simulink model "w2_warplab_trigger_proc"  (Simulink 7.7)
settings: Solver=ode45  StartTime=0.0  StopTime=1000  RelTol=1e-3
InitFcn:
  | w2_warplab_trigger_proc_init
StartFcn:
  | w2_warplab_trigger_proc_init
undefined symbols (not defined in the file or in its folder): gcbh, xlBlockLoadCallback, xlGetNormalizedPeriod
libraries: xbsIndex_r4 x819, simulink x1
(part 2 of 6)

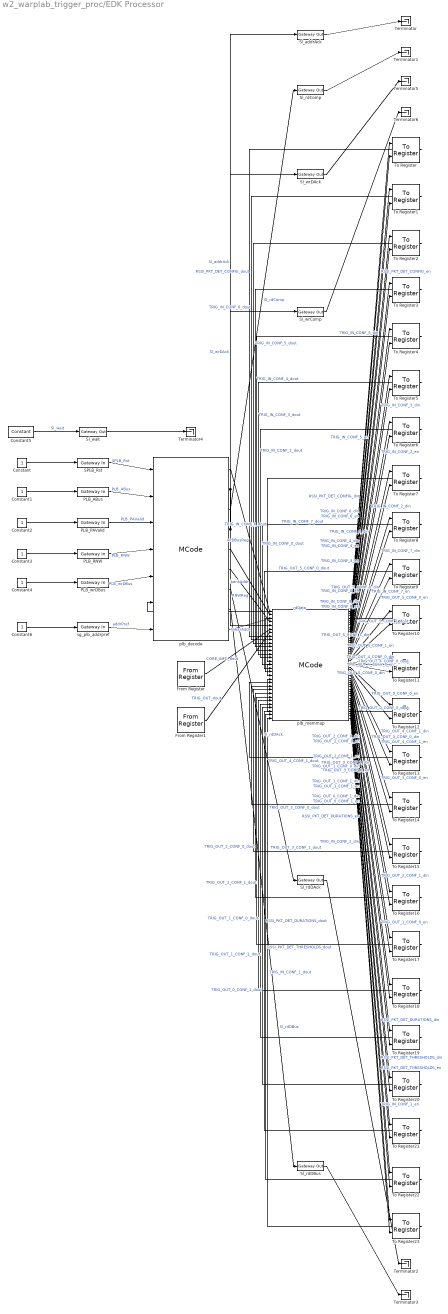
== system w2_warplab_trigger_proc/EDK Processor ==
  Constant{,1..4,6} (6 alike) : Constant
  Constant5 : xbsIndex_r4/Constant  const=0  gui_display_data_type=Fixed-point  arith_type=Unsigned  n_bits=1  bin_pt=0  preci_type=Single  exp_width=8  frac_width=24  explicit_period=on  period=xlGetNormalizedPeriod()  equ=P=C  opselect=C  inp2=PCIN>>17  opr=+  inp1=P  carry=CIN  dbl_ovrd=off  block_type=constant
  From Register : xbsIndex_r4/From Register  shared_memory_name='CORE_INFO'  init=0  period=xlGetNormalizedPeriod()  ownership=Owned and initialized elsewhere  gui_display_data_type=Fixed-point  arith_type=Unsigned  n_bits=24  bin_pt=0  preci_type=Single  dbl_ovrd=off  block_type=fromreg
      settings: AttributesFormatString=<< %<shared_memory_name> >>  infoedit="Register block that reads data to a shared memory register.  Delay of one sample period."
  From Register1 : xbsIndex_r4/From Register  shared_memory_name='TRIG_OUT'  init=0  period=xlGetNormalizedPeriod()  ownership=Owned and initialized elsewhere  gui_display_data_type=Fixed-point  arith_type=Unsigned  n_bits=6  bin_pt=0  preci_type=Single  dbl_ovrd=off  block_type=fromreg
      settings: AttributesFormatString=<< %<shared_memory_name> >>  infoedit="Register block that reads data to a shared memory register.  Delay of one sample period."
  PLB_ABus : xbsIndex_r4/Gateway In  gui_display_data_type=Fixed-point  arith_type=Unsigned  n_bits=32  bin_pt=0  preci_type=Single  exp_width=8  frac_width=24  quantization="Round  (unbiased: +/- Inf)"  overflow=Saturate  period=xlGetNormalizedPeriod()  dbl_ovrd=off  timing_constraint=None  locs_specified=off  LOCs={}  UseAsADC=off  ADCChannel='1'  inherit_from_input=off  hdl_port=on  block_type=gatewayin
      settings: sginterface={'Xilinx'=>{'jtaghwcosim'=>{'non_memory_mapped_port'=>'PLB_ABus'}},'iopad'=>{'constraint'=>'#'}}
  PLB_PAValid : xbsIndex_r4/Gateway In  gui_display_data_type=Fixed-point  arith_type=Unsigned  n_bits=1  bin_pt=0  preci_type=Single  exp_width=8  frac_width=24  quantization="Round  (unbiased: +/- Inf)"  overflow=Saturate  period=xlGetNormalizedPeriod()  dbl_ovrd=off  timing_constraint=None  locs_specified=off  LOCs={}  UseAsADC=off  ADCChannel='1'  inherit_from_input=off  hdl_port=on  block_type=gatewayin
      settings: sginterface={'Xilinx'=>{'jtaghwcosim'=>{'non_memory_mapped_port'=>'PLB_PAValid'}},'iopad'=>{'constraint'=>'#'}}
  PLB_RNW : xbsIndex_r4/Gateway In  gui_display_data_type=Fixed-point  arith_type=Unsigned  n_bits=1  bin_pt=0  preci_type=Single  exp_width=8  frac_width=24  quantization="Round  (unbiased: +/- Inf)"  overflow=Saturate  period=xlGetNormalizedPeriod()  dbl_ovrd=off  timing_constraint=None  locs_specified=off  LOCs={}  UseAsADC=off  ADCChannel='1'  inherit_from_input=off  hdl_port=on  block_type=gatewayin
      settings: sginterface={'Xilinx'=>{'jtaghwcosim'=>{'non_memory_mapped_port'=>'PLB_RNW'}},'iopad'=>{'constraint'=>'#'}}
  PLB_wrDBus : xbsIndex_r4/Gateway In  gui_display_data_type=Fixed-point  arith_type=Unsigned  n_bits=32  bin_pt=0  preci_type=Single  exp_width=8  frac_width=24  quantization="Round  (unbiased: +/- Inf)"  overflow=Saturate  period=xlGetNormalizedPeriod()  dbl_ovrd=off  timing_constraint=None  locs_specified=off  LOCs={}  UseAsADC=off  ADCChannel='1'  inherit_from_input=off  hdl_port=on  block_type=gatewayin
      settings: sginterface={'Xilinx'=>{'jtaghwcosim'=>{'non_memory_mapped_port'=>'PLB_wrDBus'}},'iopad'=>{'constraint'=>'#'}}
  SPLB_Rst : xbsIndex_r4/Gateway In  gui_display_data_type=Fixed-point  arith_type=Unsigned  n_bits=1  bin_pt=0  preci_type=Single  exp_width=8  frac_width=24  quantization="Round  (unbiased: +/- Inf)"  overflow=Saturate  period=xlGetNormalizedPeriod()  dbl_ovrd=off  timing_constraint=None  locs_specified=off  LOCs={}  UseAsADC=off  ADCChannel='1'  inherit_from_input=off  hdl_port=on  block_type=gatewayin
      settings: sginterface={'Xilinx'=>{'jtaghwcosim'=>{'non_memory_mapped_port'=>'SPLB_Rst'}},'iopad'=>{'constraint'=>'#'}}
  Sl_addrAck : xbsIndex_r4/Gateway Out  inherit_from_input=off  hdl_port=on  timing_constraint=None  locs_specified=off  LOCs={}  UseAsDAC=off  DACChannel='1'  block_type=gatewayout
      settings: sginterface={'Xilinx'=>{'jtaghwcosim'=>{'non_memory_mapped_port'=>'Sl_addrAck'}},'iopad'=>{'constraint'=>'#'}}
  Sl_rdComp : xbsIndex_r4/Gateway Out  inherit_from_input=off  hdl_port=on  timing_constraint=None  locs_specified=off  LOCs={}  UseAsDAC=off  DACChannel='1'  block_type=gatewayout
      settings: sginterface={'Xilinx'=>{'jtaghwcosim'=>{'non_memory_mapped_port'=>'Sl_rdComp'}},'iopad'=>{'constraint'=>'#'}}
  Sl_rdDAck : xbsIndex_r4/Gateway Out  inherit_from_input=off  hdl_port=on  timing_constraint=None  locs_specified=off  LOCs={}  UseAsDAC=off  DACChannel='1'  block_type=gatewayout
      settings: sginterface={'Xilinx'=>{'jtaghwcosim'=>{'non_memory_mapped_port'=>'Sl_rdDAck'}},'iopad'=>{'constraint'=>'#'}}
  Sl_rdDBus : xbsIndex_r4/Gateway Out  inherit_from_input=off  hdl_port=on  timing_constraint=None  locs_specified=off  LOCs={}  UseAsDAC=off  DACChannel='1'  block_type=gatewayout
      settings: sginterface={'Xilinx'=>{'jtaghwcosim'=>{'non_memory_mapped_port'=>'Sl_rdDBus'}},'iopad'=>{'constraint'=>'#'}}
  Sl_wait : xbsIndex_r4/Gateway Out  inherit_from_input=off  hdl_port=on  timing_constraint=None  locs_specified=off  LOCs={}  UseAsDAC=off  DACChannel='1'  block_type=gatewayout
      settings: sginterface={'Xilinx'=>{'jtaghwcosim'=>{'non_memory_mapped_port'=>'Sl_wait'}},'iopad'=>{'constraint'=>'#'}}
  Sl_wrComp : xbsIndex_r4/Gateway Out  inherit_from_input=off  hdl_port=on  timing_constraint=None  locs_specified=off  LOCs={}  UseAsDAC=off  DACChannel='1'  block_type=gatewayout
      settings: sginterface={'Xilinx'=>{'jtaghwcosim'=>{'non_memory_mapped_port'=>'Sl_wrComp'}},'iopad'=>{'constraint'=>'#'}}
  Sl_wrDAck : xbsIndex_r4/Gateway Out  inherit_from_input=off  hdl_port=on  timing_constraint=None  locs_specified=off  LOCs={}  UseAsDAC=off  DACChannel='1'  block_type=gatewayout
      settings: sginterface={'Xilinx'=>{'jtaghwcosim'=>{'non_memory_mapped_port'=>'Sl_wrDAck'}},'iopad'=>{'constraint'=>'#'}}
  Terminator{,1..6} (7 alike) : Terminator
  To Register : xbsIndex_r4/To Register  shared_memory_name='RSSI_PKT_DET_CONFIG'  init=0  ownership=Owned and initialized elsewhere  explicit_data_type=on  gui_display_data_type=Fixed-point  arith_type=Unsigned  n_bits=32  bin_pt=0  preci_type=Single  dbl_ovrd=off  block_type=toreg
      settings: AttributesFormatString=<< %<shared_memory_name> >>  infoedit="Register block that writes data to a shared memory register.  Delay of one sample period."
  To Register1 : xbsIndex_r4/To Register  shared_memory_name='TRIG_IN_CONF_6'  init=0  ownership=Owned and initialized elsewhere  explicit_data_type=on  gui_display_data_type=Fixed-point  arith_type=Unsigned  n_bits=32  bin_pt=0  preci_type=Single  dbl_ovrd=off  block_type=toreg
      settings: AttributesFormatString=<< %<shared_memory_name> >>  infoedit="Register block that writes data to a shared memory register.  Delay of one sample period."
  To Register10 : xbsIndex_r4/To Register  shared_memory_name='TRIG_OUT_5_CONF_1'  init=0  ownership=Owned and initialized elsewhere  explicit_data_type=on  gui_display_data_type=Fixed-point  arith_type=Unsigned  n_bits=32  bin_pt=0  preci_type=Single  dbl_ovrd=off  block_type=toreg
      settings: AttributesFormatString=<< %<shared_memory_name> >>  infoedit="Register block that writes data to a shared memory register.  Delay of one sample period."
  To Register11 : xbsIndex_r4/To Register  shared_memory_name='TRIG_OUT_4_CONF_0'  init=0  ownership=Owned and initialized elsewhere  explicit_data_type=on  gui_display_data_type=Fixed-point  arith_type=Unsigned  n_bits=32  bin_pt=0  preci_type=Single  dbl_ovrd=off  block_type=toreg
      settings: AttributesFormatString=<< %<shared_memory_name> >>  infoedit="Register block that writes data to a shared memory register.  Delay of one sample period."
  To Register12 : xbsIndex_r4/To Register  shared_memory_name='TRIG_OUT_0_CONF_0'  init=0  ownership=Owned and initialized elsewhere  explicit_data_type=on  gui_display_data_type=Fixed-point  arith_type=Unsigned  n_bits=32  bin_pt=0  preci_type=Single  dbl_ovrd=off  block_type=toreg
      settings: AttributesFormatString=<< %<shared_memory_name> >>  infoedit="Register block that writes data to a shared memory register.  Delay of one sample period."
  To Register13 : xbsIndex_r4/To Register  shared_memory_name='TRIG_OUT_4_CONF_1'  init=0  ownership=Owned and initialized elsewhere  explicit_data_type=on  gui_display_data_type=Fixed-point  arith_type=Unsigned  n_bits=32  bin_pt=0  preci_type=Single  dbl_ovrd=off  block_type=toreg
      settings: AttributesFormatString=<< %<shared_memory_name> >>  infoedit="Register block that writes data to a shared memory register.  Delay of one sample period."
  To Register14 : xbsIndex_r4/To Register  shared_memory_name='TRIG_OUT_3_CONF_0'  init=0  ownership=Owned and initialized elsewhere  explicit_data_type=on  gui_display_data_type=Fixed-point  arith_type=Unsigned  n_bits=32  bin_pt=0  preci_type=Single  dbl_ovrd=off  block_type=toreg
      settings: AttributesFormatString=<< %<shared_memory_name> >>  infoedit="Register block that writes data to a shared memory register.  Delay of one sample period."
  To Register15 : xbsIndex_r4/To Register  shared_memory_name='TRIG_OUT_3_CONF_1'  init=0  ownership=Owned and initialized elsewhere  explicit_data_type=on  gui_display_data_type=Fixed-point  arith_type=Unsigned  n_bits=32  bin_pt=0  preci_type=Single  dbl_ovrd=off  block_type=toreg
      settings: AttributesFormatString=<< %<shared_memory_name> >>  infoedit="Register block that writes data to a shared memory register.  Delay of one sample period."
  To Register16 : xbsIndex_r4/To Register  shared_memory_name='TRIG_OUT_2_CONF_0'  init=0  ownership=Owned and initialized elsewhere  explicit_data_type=on  gui_display_data_type=Fixed-point  arith_type=Unsigned  n_bits=32  bin_pt=0  preci_type=Single  dbl_ovrd=off  block_type=toreg
      settings: AttributesFormatString=<< %<shared_memory_name> >>  infoedit="Register block that writes data to a shared memory register.  Delay of one sample period."
  To Register17 : xbsIndex_r4/To Register  shared_memory_name='TRIG_OUT_2_CONF_1'  init=0  ownership=Owned and initialized elsewhere  explicit_data_type=on  gui_display_data_type=Fixed-point  arith_type=Unsigned  n_bits=32  bin_pt=0  preci_type=Single  dbl_ovrd=off  block_type=toreg
      settings: AttributesFormatString=<< %<shared_memory_name> >>  infoedit="Register block that writes data to a shared memory register.  Delay of one sample period."
  To Register18 : xbsIndex_r4/To Register  shared_memory_name='TRIG_OUT_1_CONF_0'  init=0  ownership=Owned and initialized elsewhere  explicit_data_type=on  gui_display_data_type=Fixed-point  arith_type=Unsigned  n_bits=32  bin_pt=0  preci_type=Single  dbl_ovrd=off  block_type=toreg
      settings: AttributesFormatString=<< %<shared_memory_name> >>  infoedit="Register block that writes data to a shared memory register.  Delay of one sample period."
  To Register19 : xbsIndex_r4/To Register  shared_memory_name='TRIG_OUT_1_CONF_1'  init=0  ownership=Owned and initialized elsewhere  explicit_data_type=on  gui_display_data_type=Fixed-point  arith_type=Unsigned  n_bits=32  bin_pt=0  preci_type=Single  dbl_ovrd=off  block_type=toreg
      settings: AttributesFormatString=<< %<shared_memory_name> >>  infoedit="Register block that writes data to a shared memory register.  Delay of one sample period."
  To Register2 : xbsIndex_r4/To Register  shared_memory_name='TRIG_IN_CONF_5'  init=0  ownership=Owned and initialized elsewhere  explicit_data_type=on  gui_display_data_type=Fixed-point  arith_type=Unsigned  n_bits=32  bin_pt=0  preci_type=Single  dbl_ovrd=off  block_type=toreg
      settings: AttributesFormatString=<< %<shared_memory_name> >>  infoedit="Register block that writes data to a shared memory register.  Delay of one sample period."
  To Register20 : xbsIndex_r4/To Register  shared_memory_name='TRIG_OUT_0_CONF_1'  init=0  ownership=Owned and initialized elsewhere  explicit_data_type=on  gui_display_data_type=Fixed-point  arith_type=Unsigned  n_bits=32  bin_pt=0  preci_type=Single  dbl_ovrd=off  block_type=toreg
      settings: AttributesFormatString=<< %<shared_memory_name> >>  infoedit="Register block that writes data to a shared memory register.  Delay of one sample period."
  To Register21 : xbsIndex_r4/To Register  shared_memory_name='RSSI_PKT_DET_DURATIONS'  init=0  ownership=Owned and initialized elsewhere  explicit_data_type=on  gui_display_data_type=Fixed-point  arith_type=Unsigned  n_bits=32  bin_pt=0  preci_type=Single  dbl_ovrd=off  block_type=toreg
      settings: AttributesFormatString=<< %<shared_memory_name> >>  infoedit="Register block that writes data to a shared memory register.  Delay of one sample period."
  To Register22 : xbsIndex_r4/To Register  shared_memory_name='RSSI_PKT_DET_THRESHOLDS'  init=0  ownership=Owned and initialized elsewhere  explicit_data_type=on  gui_display_data_type=Fixed-point  arith_type=Unsigned  n_bits=32  bin_pt=0  preci_type=Single  dbl_ovrd=off  block_type=toreg
      settings: AttributesFormatString=<< %<shared_memory_name> >>  infoedit="Register block that writes data to a shared memory register.  Delay of one sample period."
  To Register23 : xbsIndex_r4/To Register  shared_memory_name='TRIG_IN_CONF_1'  init=0  ownership=Owned and initialized elsewhere  explicit_data_type=on  gui_display_data_type=Fixed-point  arith_type=Unsigned  n_bits=32  bin_pt=0  preci_type=Single  dbl_ovrd=off  block_type=toreg
      settings: AttributesFormatString=<< %<shared_memory_name> >>  infoedit="Register block that writes data to a shared memory register.  Delay of one sample period."
  To Register3 : xbsIndex_r4/To Register  shared_memory_name='TRIG_IN_CONF_4'  init=0  ownership=Owned and initialized elsewhere  explicit_data_type=on  gui_display_data_type=Fixed-point  arith_type=Unsigned  n_bits=32  bin_pt=0  preci_type=Single  dbl_ovrd=off  block_type=toreg
      settings: AttributesFormatString=<< %<shared_memory_name> >>  infoedit="Register block that writes data to a shared memory register.  Delay of one sample period."
  To Register4 : xbsIndex_r4/To Register  shared_memory_name='TRIG_IN_CONF_3'  init=0  ownership=Owned and initialized elsewhere  explicit_data_type=on  gui_display_data_type=Fixed-point  arith_type=Unsigned  n_bits=32  bin_pt=0  preci_type=Single  dbl_ovrd=off  block_type=toreg
      settings: AttributesFormatString=<< %<shared_memory_name> >>  infoedit="Register block that writes data to a shared memory register.  Delay of one sample period."
  To Register5 : xbsIndex_r4/To Register  shared_memory_name='TRIG_IN_CONF_2'  init=0  ownership=Owned and initialized elsewhere  explicit_data_type=on  gui_display_data_type=Fixed-point  arith_type=Unsigned  n_bits=32  bin_pt=0  preci_type=Single  dbl_ovrd=off  block_type=toreg
      settings: AttributesFormatString=<< %<shared_memory_name> >>  infoedit="Register block that writes data to a shared memory register.  Delay of one sample period."
  To Register6 : xbsIndex_r4/To Register  shared_memory_name='TRIG_IN_CONF_0'  init=0  ownership=Owned and initialized elsewhere  explicit_data_type=on  gui_display_data_type=Fixed-point  arith_type=Unsigned  n_bits=32  bin_pt=0  preci_type=Single  dbl_ovrd=off  block_type=toreg
      settings: AttributesFormatString=<< %<shared_memory_name> >>  infoedit="Register block that writes data to a shared memory register.  Delay of one sample period."
  To Register7 : xbsIndex_r4/To Register  shared_memory_name='TRIG_IN_CONF_8'  init=0  ownership=Owned and initialized elsewhere  explicit_data_type=on  gui_display_data_type=Fixed-point  arith_type=Unsigned  n_bits=32  bin_pt=0  preci_type=Single  dbl_ovrd=off  block_type=toreg
      settings: AttributesFormatString=<< %<shared_memory_name> >>  infoedit="Register block that writes data to a shared memory register.  Delay of one sample period."
  To Register8 : xbsIndex_r4/To Register  shared_memory_name='TRIG_IN_CONF_7'  init=0  ownership=Owned and initialized elsewhere  explicit_data_type=on  gui_display_data_type=Fixed-point  arith_type=Unsigned  n_bits=32  bin_pt=0  preci_type=Single  dbl_ovrd=off  block_type=toreg
      settings: AttributesFormatString=<< %<shared_memory_name> >>  infoedit="Register block that writes data to a shared memory register.  Delay of one sample period."
  To Register9 : xbsIndex_r4/To Register  shared_memory_name='TRIG_OUT_5_CONF_0'  init=0  ownership=Owned and initialized elsewhere  explicit_data_type=on  gui_display_data_type=Fixed-point  arith_type=Unsigned  n_bits=32  bin_pt=0  preci_type=Single  dbl_ovrd=off  block_type=toreg
      settings: AttributesFormatString=<< %<shared_memory_name> >>  infoedit="Register block that writes data to a shared memory register.  Delay of one sample period."
  plb_decode : xbsIndex_r4/MCode  mfname=xlmax  explicit_period=off  period=1  dbl_ovrd=off  enable_stdout=off  enable_debug=off  mfilecontent=|  suppress_output=on  defparams={}  hide_port_list={}  block_type=mcode
      | function [wrDBusReg, addrAck, rdComp, wrDAck, bankAddr, RNWReg, rdDAck, rdDBus, linearAddr] = plb_bus_decode(plbRst, plbABus, plbPAValid, plbRNW, plbWrDBus, rdData, addrPref)
      | 
      | % constant variables (TODO: should pass from outside)
      | ADDRPREF_LEN = 20;
      | BANKADDR_LEN = 2;
      | LINEARADDR_LEN = 8;
      | ABUS_LEN = 32;
      | DBUS_LEN = 32;
      | 
      | % declare and initialize persistent variables
      | % register input bus signals
      | persistent plbRstReg_, plbRstReg_ = xl_state(0, {xlBoolean});
      | persistent plbABusReg_, plbABusReg_ = xl_state(0, {xlUnsigned, ABUS_LEN, 0});
      | persistent plbPAValidReg_, plbPAValidReg_ = xl_state(0, {xlBoolean});
      | persistent plbRNWReg_, plbRNWReg_ = xl_state(0, {xlUnsigned, 1, 0});
      | persistent plbWrDBusReg_, plbWrDBusReg_ = xl_state(0, {xlUnsigned, DBUS_LEN, 0});
      | 
      | % ===== rest of the outputs =====
      | 
      | bankAddr   = xl_slice(plbABusReg_, 2+BANKADDR_LEN+LINEARADDR_LEN-1, 2+LINEARADDR_LEN);
      | linearAddr = xl_slice(plbABusReg_, 2+LINEARADDR_LEN-1, 2);
      | RNWReg = plbRNWReg_;
      | wrDBusReg = plbWrDBusReg_;
      | 
      | % ===== p_select =====
      | 
      | % register PAValid
      | persistent aValidReg, aValidReg = xl_state(0, {xlBoolean});
      | aValidReg = plbPAValidReg_;
      | 
      | % extract and register the address prefix
      | addrPref_in = xl_slice(plbABusReg_, xl_nbits(plbABusReg_)-1, xl_nbits(plbABusReg_)-ADDRPREF_LEN);
      | if addrPref_in == addrPref
      |     ps1 = true;
      | else 
      |     ps1 = false;
      | end 
      | 
      | persistent ps1Reg, ps1Reg = xl_state(0, ps1);
      | ps1Reg = ps1;
      | 
      | ps = xl_and(ps1Reg, aValidReg);
      | 
      | % ===== addrAck =====
      | 
      | % register ps
      | persistent psReg, psReg = xl_state(0, ps);
      | 
      | addrAck = xfix({xlUnsigned, 1, 0}, xl_and(xl_not(plbRstReg_), ps, xl_not(psReg)));
      | 
      | psReg = ps;
      | 
      | % ===== rdComp, rd/wr DAck =====
      |  
      | rdComp1 = xfix({xlUnsigned, 1, 0}, xl_and(addrAck, RNWReg));
      | 
      | NUM_rdCompDelay = 3;
      | persistent rdCompDelay, rdCompDelay = xl_state(zeros(1, NUM_rdCompDelay), rdComp1, NUM_rdCompDelay);
      | rdComp2 = rdCompDelay.back;
      | rdCompDelay.push_front_pop_back(rdComp1);
      | 
      | persistent rdCompReg, rdCompReg = xl_state(0, rdComp1);
      | rdComp = rdCompReg;
      | rdCompReg = rdComp2;
      | 
      | persistent rdDAckReg, rdDAckReg = xl_state(0, rdComp1);
      | rdDAck = rdDAckReg;
      | rdDAckReg = rdComp;
      | 
      | persistent wrDAckReg, wrDAckReg = xl_state(0, addrAck);
      | wrDAck = wrDAckReg;
      | wrDAckReg = xl_and(addrAck, xl_not(RNWReg));
      | 
      | % ===== rdDBus =====
      | 
      | rdSel = xl_or(rdComp2, rdComp);
      | 
      | if rdSel == 1
      |     rdDBus1 = rdData;
      | else
      |     rdDBus1 = 0;
      | end % if
      | 
      | persistent rdDBusReg, rdDBusReg = xl_state(0, rdDBus1);
      | rdDBus = rdDBusReg;
      | rdDBusReg = rdDBus1;
      | 
      | % rdDBus = xl_concat(rdDBus32, rdDBus32);
      | % rdDBus = rdDBus32;
      | 
      | % ===== update the persistent variables =====
      | 
      | plbRstReg_ = plbRst;
      | plbABusReg_ = plbABus;
      | plbPAValidReg_ = plbPAValid;
      | plbRNWReg_ = plbRNW;
      | plbWrDBusReg_ = xl_slice(plbWrDBus, DBUS_LEN-1, 0);
  plb_memmap : xbsIndex_r4/MCode  mfname=xlmax  explicit_period=off  period=1  dbl_ovrd=off  enable_stdout=off  enable_debug=off  mfilecontent=|  suppress_output=on  defparams={}  hide_port_list={}  block_type=mcode
      | function [read_bank_out, sm_RSSI_PKT_DET_CONFIG_din, sm_RSSI_PKT_DET_CONFIG_en, sm_TRIG_IN_CONF_6_din, sm_TRIG_IN_CONF_6_en, sm_TRIG_IN_CONF_5_din, sm_TRIG_IN_CONF_5_en, sm_TRIG_IN_CONF_4_din, sm_TRIG_IN_CONF_4_en, sm_TRIG_IN_CONF_3_din, sm_TRIG_IN_CONF_3_en, sm_TRIG_IN_CONF_2_din, sm_TRIG_IN_CONF_2_en, sm_TRIG_IN_CONF_0_din, sm_TRIG_IN_CONF_0_en, sm_TRIG_IN_CONF_8_din, sm_TRIG_IN_CONF_8_en, sm_TRIG_IN_CONF_7_din, sm_TRIG_IN_CONF_7_en, sm_TRIG_OUT_5_CONF_0_din, sm_TRIG_OUT_5_CONF_0_en, sm_TRIG_OUT_5_CONF_1_din, sm_TRIG_OUT_5_CONF_1_en, sm_TRIG_OUT_4_CONF_0_din, sm_TRIG_OUT_4_CONF_0_en, sm_TRIG_OUT_0_CONF_0_din, sm_TRIG_OUT_0_CONF_0_en, sm_TRIG_OUT_4_CONF_1_din, sm_TRIG_OUT_4_CONF_1_en, sm_TRIG_OUT_3_CONF_0_din, sm_TRIG_OUT_3_CONF_0_en, sm_TRIG_OUT_3_CONF_1_din, sm_TRIG_OUT_3_CONF_1_en, sm_TRIG_OUT_2_CONF_0_din, sm_TRIG_OUT_2_CONF_0_en, sm_TRIG_OUT_2_CONF_1_din, sm_TRIG_OUT_2_CONF_1_en, sm_TRIG_OUT_1_CONF_0_din, sm_TRIG_OUT_1_CONF_0_en, sm_TRIG_OUT_1_CONF_1_din, sm_TRIG_OUT_1_CONF_1_en, sm_TRIG_OUT_0_CONF_1_din, sm_TRIG_OUT_0_CONF_1_en, sm_RSSI_PKT_DET_DURATIONS_din, sm_RSSI_PKT_DET_DURATIONS_en, sm_RSSI_PKT_DET_THRESHOLDS_din, sm_RSSI_PKT_DET_THRESHOLDS_en, sm_TRIG_IN_CONF_1_din, sm_TRIG_IN_CONF_1_en] = plb_memmap(wrDBus, bankAddr, linearAddr, RNWReg, addrAck, sm_CORE_INFO, sm_TRIG_OUT, sm_RSSI_PKT_DET_CONFIG, sm_TRIG_IN_CONF_6, sm_TRIG_IN_CONF_5, sm_TRIG_IN_CONF_4, sm_TRIG_IN_CONF_3, sm_TRIG_IN_CONF_2, sm_TRIG_IN_CONF_0, sm_TRIG_IN_CONF_8, sm_TRIG_IN_CONF_7, sm_TRIG_OUT_5_CONF_0, sm_TRIG_OUT_5_CONF_1, sm_TRIG_OUT_4_CONF_0, sm_TRIG_OUT_0_CONF_0, sm_TRIG_OUT_4_CONF_1, sm_TRIG_OUT_3_CONF_0, sm_TRIG_OUT_3_CONF_1, sm_TRIG_OUT_2_CONF_0, sm_TRIG_OUT_2_CONF_1, sm_TRIG_OUT_1_CONF_0, sm_TRIG_OUT_1_CONF_1, sm_TRIG_OUT_0_CONF_1, sm_RSSI_PKT_DET_DURATIONS, sm_RSSI_PKT_DET_THRESHOLDS, sm_TRIG_IN_CONF_1)
      | 
      | 
      | % connvert the input data to UFix_32_0 (the bus data type)
      | % 'From Register' blocks
      | % sm_CORE_INFO_bus = xfix({xlUnsigned, 32, 0}, 0);
      | sm_CORE_INFO_bus = xl_force(sm_CORE_INFO, xlUnsigned, 0);
      | 
      | % sm_TRIG_OUT_bus = xfix({xlUnsigned, 32, 0}, 0);
      | sm_TRIG_OUT_bus = xl_force(sm_TRIG_OUT, xlUnsigned, 0);
      | 
      | % 'To Register' blocks
      | 
      | % sm_RSSI_PKT_DET_CONFIG_dout = xfix({xlUnsigned, 32, 0}, 0);
      | sm_RSSI_PKT_DET_CONFIG_dout = xl_force(sm_RSSI_PKT_DET_CONFIG, xlUnsigned, 0);
      | 
      | % sm_TRIG_IN_CONF_6_dout = xfix({xlUnsigned, 32, 0}, 0);
      | sm_TRIG_IN_CONF_6_dout = xl_force(sm_TRIG_IN_CONF_6, xlUnsigned, 0);
      | 
      | % sm_TRIG_IN_CONF_5_dout = xfix({xlUnsigned, 32, 0}, 0);
      | sm_TRIG_IN_CONF_5_dout = xl_force(sm_TRIG_IN_CONF_5, xlUnsigned, 0);
      | 
      | % sm_TRIG_IN_CONF_4_dout = xfix({xlUnsigned, 32, 0}, 0);
      | sm_TRIG_IN_CONF_4_dout = xl_force(sm_TRIG_IN_CONF_4, xlUnsigned, 0);
      | 
      | % sm_TRIG_IN_CONF_3_dout = xfix({xlUnsigned, 32, 0}, 0);
      | sm_TRIG_IN_CONF_3_dout = xl_force(sm_TRIG_IN_CONF_3, xlUnsigned, 0);
      | 
      | % sm_TRIG_IN_CONF_2_dout = xfix({xlUnsigned, 32, 0}, 0);
      | sm_TRIG_IN_CONF_2_dout = xl_force(sm_TRIG_IN_CONF_2, xlUnsigned, 0);
      | 
      | % sm_TRIG_IN_CONF_0_dout = xfix({xlUnsigned, 32, 0}, 0);
      | sm_TRIG_IN_CONF_0_dout = xl_force(sm_TRIG_IN_CONF_0, xlUnsigned, 0);
      | 
      | % sm_TRIG_IN_CONF_8_dout = xfix({xlUnsigned, 32, 0}, 0);
      | sm_TRIG_IN_CONF_8_dout = xl_force(sm_TRIG_IN_CONF_8, xlUnsigned, 0);
      | 
      | % sm_TRIG_IN_CONF_7_dout = xfix({xlUnsigned, 32, 0}, 0);
      | sm_TRIG_IN_CONF_7_dout = xl_force(sm_TRIG_IN_CONF_7, xlUnsigned, 0);
      | 
      | % sm_TRIG_OUT_5_CONF_0_dout = xfix({xlUnsigned, 32, 0}, 0);
      | sm_TRIG_OUT_5_CONF_0_dout = xl_force(sm_TRIG_OUT_5_CONF_0, xlUnsigned, 0);
      | 
      | % sm_TRIG_OUT_5_CONF_1_dout = xfix({xlUnsigned, 32, 0}, 0);
      | sm_TRIG_OUT_5_CONF_1_dout = xl_force(sm_TRIG_OUT_5_CONF_1, xlUnsigned, 0);
      | 
      | % sm_TRIG_OUT_4_CONF_0_dout = xfix({xlUnsigned, 32, 0}, 0);
      | sm_TRIG_OUT_4_CONF_0_dout = xl_force(sm_TRIG_OUT_4_CONF_0, xlUnsigned, 0);
      | 
      | % sm_TRIG_OUT_0_CONF_0_dout = xfix({xlUnsigned, 32, 0}, 0);
      | sm_TRIG_OUT_0_CONF_0_dout = xl_force(sm_TRIG_OUT_0_CONF_0, xlUnsigned, 0);
      | 
      | % sm_TRIG_OUT_4_CONF_1_dout = xfix({xlUnsigned, 32, 0}, 0);
      | sm_TRIG_OUT_4_CONF_1_dout = xl_force(sm_TRIG_OUT_4_CONF_1, xlUnsigned, 0);
      | 
      | % sm_TRIG_OUT_3_CONF_0_dout = xfix({xlUnsigned, 32, 0}, 0);
      | sm_TRIG_OUT_3_CONF_0_dout = xl_force(sm_TRIG_OUT_3_CONF_0, xlUnsigned, 0);
      | 
      | % sm_TRIG_OUT_3_CONF_1_dout = xfix({xlUnsigned, 32, 0}, 0);
      | sm_TRIG_OUT_3_CONF_1_dout = xl_force(sm_TRIG_OUT_3_CONF_1, xlUnsigned, 0);
      | 
      | % sm_TRIG_OUT_2_CONF_0_dout = xfix({xlUnsigned, 32, 0}, 0);
      | sm_TRIG_OUT_2_CONF_0_dout = xl_force(sm_TRIG_OUT_2_CONF_0, xlUnsigned, 0);
      | 
      | % sm_TRIG_OUT_2_CONF_1_dout = xfix({xlUnsigned, 32, 0}, 0);
      | sm_TRIG_OUT_2_CONF_1_dout = xl_force(sm_TRIG_OUT_2_CONF_1, xlUnsigned, 0);
      | 
      | % sm_TRIG_OUT_1_CONF_0_dout = xfix({xlUnsigned, 32, 0}, 0);
      | sm_TRIG_OUT_1_CONF_0_dout = xl_force(sm_TRIG_OUT_1_CONF_0, xlUnsigned, 0);
      | 
      | % sm_TRIG_OUT_1_CONF_1_dout = xfix({xlUnsigned, 32, 0}, 0);
      | sm_TRIG_OUT_1_CONF_1_dout = xl_force(sm_TRIG_OUT_1_CONF_1, xlUnsigned, 0);
      | 
      | % sm_TRIG_OUT_0_CONF_1_dout = xfix({xlUnsigned, 32, 0}, 0);
      | sm_TRIG_OUT_0_CONF_1_dout = xl_force(sm_TRIG_OUT_0_CONF_1, xlUnsigned, 0);
      | 
      | % sm_RSSI_PKT_DET_DURATIONS_dout = xfix({xlUnsigned, 32, 0}, 0);
      | sm_RSSI_PKT_DET_DURATIONS_dout = xl_force(sm_RSSI_PKT_DET_DURATIONS, xlUnsigned, 0);
      | 
      | % sm_RSSI_PKT_DET_THRESHOLDS_dout = xfix({xlUnsigned, 32, 0}, 0);
      | sm_RSSI_PKT_DET_THRESHOLDS_dout = xl_force(sm_RSSI_PKT_DET_THRESHOLDS, xlUnsigned, 0);
      | 
      | % sm_TRIG_IN_CONF_1_dout = xfix({xlUnsigned, 32, 0}, 0);
      | sm_TRIG_IN_CONF_1_dout = xl_force(sm_TRIG_IN_CONF_1, xlUnsigned, 0);
      | 
      | 
      | % 'From FIFO' blocks
      | % 'To FIFO' blocks
      | % 'Shared Memory' blocks
      | 
      | % 'dout' ports of 'From Register' blocks
      | 
      | % registered register mux output
      | persistent reg_bank_out_reg; reg_bank_out_reg = xl_state(0, {xlUnsigned, 32, 0});
      | reg_bank_out = reg_bank_out_reg;
      | 
      | if linearAddr == 24
      |     reg_bank_out_reg = sm_CORE_INFO_bus;
      | elseif linearAddr == 25
      |     reg_bank_out_reg = sm_TRIG_OUT_bus;
      | elseif linearAddr == 0
      |     reg_bank_out_reg = sm_RSSI_PKT_DET_CONFIG_dout;
      | elseif linearAddr == 1
      |     reg_bank_out_reg = sm_TRIG_IN_CONF_6_dout;
      | elseif linearAddr == 2
      |     reg_bank_out_reg = sm_TRIG_IN_CONF_5_dout;
      | elseif linearAddr == 3
      |     reg_bank_out_reg = sm_TRIG_IN_CONF_4_dout;
      | elseif linearAddr == 4
      |     reg_bank_out_reg = sm_TRIG_IN_CONF_3_dout;
      | elseif linearAddr == 5
      |     reg_bank_out_reg = sm_TRIG_IN_CONF_2_dout;
      | elseif linearAddr == 6
      |     reg_bank_out_reg = sm_TRIG_IN_CONF_0_dout;
      | elseif linearAddr == 7
      |     reg_bank_out_reg = sm_TRIG_IN_CONF_8_dout;
      | elseif linearAddr == 8
      |     reg_bank_out_reg = sm_TRIG_IN_CONF_7_dout;
      | elseif linearAddr == 9
      |     reg_bank_out_reg = sm_TRIG_OUT_5_CONF_0_dout;
      | elseif linearAddr == 10
      |     reg_bank_out_reg = sm_TRIG_OUT_5_CONF_1_dout;
      | elseif linearAddr == 11
      |     reg_bank_out_reg = sm_TRIG_OUT_4_CONF_0_dout;
      | elseif linearAddr == 12
      |     reg_bank_out_reg = sm_TRIG_OUT_0_CONF_0_dout;
      | elseif linearAddr == 13
      |     reg_bank_out_reg = sm_TRIG_OUT_4_CONF_1_dout;
      | elseif linearAddr == 14
      |     reg_bank_out_reg = sm_TRIG_OUT_3_CONF_0_dout;
      | elseif linearAddr == 15
      |     reg_bank_out_reg = sm_TRIG_OUT_3_CONF_1_dout;
      | elseif linearAddr == 16
      |     reg_bank_out_reg = sm_TRIG_OUT_2_CONF_0_dout;
      | elseif linearAddr == 17
      |     reg_bank_out_reg = sm_TRIG_OUT_2_CONF_1_dout;
      | elseif linearAddr == 18
      |     reg_bank_out_reg = sm_TRIG_OUT_1_CONF_0_dout;
      | elseif linearAddr == 19
      |     reg_bank_out_reg = sm_TRIG_OUT_1_CONF_1_dout;
      | elseif linearAddr == 20
      |     reg_bank_out_reg = sm_TRIG_OUT_0_CONF_1_dout;
      | elseif linearAddr == 21
      |     reg_bank_out_reg = sm_RSSI_PKT_DET_DURATIONS_dout;
      | elseif linearAddr == 22
      |     reg_bank_out_reg = sm_RSSI_PKT_DET_THRESHOLDS_dout;
      | elseif linearAddr == 23
      |     reg_bank_out_reg = sm_TRIG_IN_CONF_1_dout;
      | 
      | end
      | 
      | 
      | % 'From FIFO' and 'To FIFO' blocks
      | 
      | 
      | 
      | 
      | 
      | opCode = xl_concat(addrAck, RNWReg, bankAddr, linearAddr);
      | 
      | % 'Shared Memory' blocks
      | 
      | 
      | 
      | 
      | 
      | % 'din' ports of 'Shared Memory' blocks
      | 
      | 
      | % 'we' ports of 'Shared Memory' blocks
      | 
      | 
      | % 'addr' ports of 'Shared Memory' blocks
      | 
      | 
      | % 're' ports of 'From FIFO' blocks
      | 
      | 
      | % 'en' ports of 'To Register' blocks
      | if opCode == xl_concat(xfix({xlUnsigned, 4, 0}, 10), ...
      |                        xfix({xlUnsigned, xl_nbits(linearAddr), 0}, 0))
      |     sm_RSSI_PKT_DET_CONFIG_en = true;
      | else
      |     sm_RSSI_PKT_DET_CONFIG_en = false;
      | end
      | if opCode == xl_concat(xfix({xlUnsigned, 4, 0}, 10), ...
      |                        xfix({xlUnsigned, xl_nbits(linearAddr), 0}, 1))
      |     sm_TRIG_IN_CONF_6_en = true;
      | else
      |     sm_TRIG_IN_CONF_6_en = false;
      | end
      | if opCode == xl_concat(xfix({xlUnsigned, 4, 0}, 10), ...
      |                        xfix({xlUnsigned, xl_nbits(linearAddr), 0}, 2))
      |     sm_TRIG_IN_CONF_5_en = true;
      | else
      |     sm_TRIG_IN_CONF_5_en = false;
      | end
      | if opCode == xl_concat(xfix({xlUnsigned, 4, 0}, 10), ...
      |                        xfix({xlUnsigned, xl_nbits(linearAddr), 0}, 3))
      |     sm_TRIG_IN_CONF_4_en = true;
      | else
      |     sm_TRIG_IN_CONF_4_en = false;
      | end
      | if opCode == xl_concat(xfix({xlUnsigned, 4, 0}, 10), ...
      |                        xfix({xlUnsigned, xl_nbits(linearAddr), 0}, 4))
      |     sm_TRIG_IN_CONF_3_en = true;
      | else
      |     sm_TRIG_IN_CONF_3_en = false;
      | end
      | if opCode == xl_concat(xfix({xlUnsigned, 4, 0}, 10), ...
      |                        xfix({xlUnsigned, xl_nbits(linearAddr), 0}, 5))
      |     sm_TRIG_IN_CONF_2_en = true;
      | else
      |     sm_TRIG_IN_CONF_2_en = false;
      | end
      | if opCode == xl_concat(xfix({xlUnsigned, 4, 0}, 10), ...
      |                        xfix({xlUnsigned, xl_nbits(linearAddr), 0}, 6))
      |     sm_TRIG_IN_CONF_0_en = true;
      | else
      |     sm_TRIG_IN_CONF_0_en = false;
      | end
      | if opCode == xl_concat(xfix({xlUnsigned, 4, 0}, 10), ...
      |                        xfix({xlUnsigned, xl_nbits(linearAddr), 0}, 7))
      |     sm_TRIG_IN_CONF_8_en = true;
      | else
      |     sm_TRIG_IN_CONF_8_en = false;
      | end
      | if opCode == xl_concat(xfix({xlUnsigned, 4, 0}, 10), ...
      |                        xfix({xlUnsigned, xl_nbits(linearAddr), 0}, 8))
      |     sm_TRIG_IN_CONF_7_en = true;
      | else
      |     sm_TRIG_IN_CONF_7_en = false;
      | end
      | if opCode == xl_concat(xfix({xlUnsigned, 4, 0}, 10), ...
      |                        xfix({xlUnsigned, xl_nbits(linearAddr), 0}, 9))
      |     sm_TRIG_OUT_5_CONF_0_en = true;
      | else
      |     sm_TRIG_OUT_5_CONF_0_en = false;
      | end
      | if opCode == xl_concat(xfix({xlUnsigned, 4, 0}, 10), ...
      |                        xfix({xlUnsigned, xl_nbits(linearAddr), 0}, 10))
      |     sm_TRIG_OUT_5_CONF_1_en = true;
      | else
      |     sm_TRIG_OUT_5_CONF_1_en = false;
      | end
      | if opCode == xl_concat(xfix({xlUnsigned, 4, 0}, 10), ...
      |                        xfix({xlUnsigned, xl_nbits(linearAddr), 0}, 11))
      |     sm_TRIG_OUT_4_CONF_0_en = true;
      | else
      |     sm_TRIG_OUT_4_CONF_0_en = false;
      | end
      | if opCode == xl_concat(xfix({xlUnsigned, 4, 0}, 10), ...
      |                        xfix({xlUnsigned, xl_nbits(linearAddr), 0}, 12))
      |     sm_TRIG_OUT_0_CONF_0_en = true;
      | else
      |     sm_TRIG_OUT_0_CONF_0_en = false;
      | end
      | if opCode == xl_concat(xfix({xlUnsigned, 4, 0}, 10), ...
      |                        xfix({xlUnsigned, xl_nbits(linearAddr), 0}, 13))
      |     sm_TRIG_OUT_4_CONF_1_en = true;
      | else
      |     sm_TRIG_OUT_4_CONF_1_en = false;
      | end
      | if opCode == xl_concat(xfix({xlUnsigned, 4, 0}, 10), ...
      |                        xfix({xlUnsigned, xl_nbits(linearAddr), 0}, 14))
      |     sm_TRIG_OUT_3_CONF_0_en = true;
      | else
      |     sm_TRIG_OUT_3_CONF_0_en = false;
      | end
      | if opCode == xl_concat(xfix({xlUnsigned, 4, 0}, 10), ...
      |                        xfix({xlUnsigned, xl_nbits(linearAddr), 0}, 15))
      |     sm_TRIG_OUT_3_CONF_1_en = true;
      | else
      |     sm_TRIG_OUT_3_CONF_1_en = false;
      | end
      | if opCode == xl_concat(xfix({xlUnsigned, 4, 0}, 10), ...
      |                        xfix({xlUnsigned, xl_nbits(linearAddr), 0}, 16))
      |     sm_TRIG_OUT_2_CONF_0_en = true;
      | else
      |     sm_TRIG_OUT_2_CONF_0_en = false;
      | end
      | if opCode == xl_concat(xfix({xlUnsigned, 4, 0}, 10), ...
      |                        xfix({xlUnsigned, xl_nbits(linearAddr), 0}, 17))
      |     sm_TRIG_OUT_2_CONF_1_en = true;
      | else
      |     sm_TRIG_OUT_2_CONF_1_en = false;
      | end
      | if opCode == xl_concat(xfix({xlUnsigned, 4, 0}, 10), ...
      |                        xfix({xlUnsigned, xl_nbits(linearAddr), 0}, 18))
      |     sm_TRIG_OUT_1_CONF_0_en = true;
      | else
      |     sm_TRIG_OUT_1_CONF_0_en = false;
      | end
      | if opCode == xl_concat(xfix({xlUnsigned, 4, 0}, 10), ...
      |                        xfix({xlUnsigned, xl_nbits(linearAddr), 0}, 19))
      |     sm_TRIG_OUT_1_CONF_1_en = true;
      | else
      |     sm_TRIG_OUT_1_CONF_1_en = false;
      | end
      | if opCode == xl_concat(xfix({xlUnsigned, 4, 0}, 10), ...
      |                        xfix({xlUnsigned, xl_nbits(linearAddr), 0}, 20))
      |     sm_TRIG_OUT_0_CONF_1_en = true;
      | else
      |     sm_TRIG_OUT_0_CONF_1_en = false;
      | end
      | if opCode == xl_concat(xfix({xlUnsigned, 4, 0}, 10), ...
      |                        xfix({xlUnsigned, xl_nbits(linearAddr), 0}, 21))
      |     sm_RSSI_PKT_DET_DURATIONS_en = true;
      | else
      |     sm_RSSI_PKT_DET_DURATIONS_en = false;
      | end
      | if opCode == xl_concat(xfix({xlUnsigned, 4, 0}, 10), ...
      |                        xfix({xlUnsigned, xl_nbits(linearAddr), 0}, 22))
      |     sm_RSSI_PKT_DET_THRESHOLDS_en = true;
      | else
      |     sm_RSSI_PKT_DET_THRESHOLDS_en = false;
      | end
      | if opCode == xl_concat(xfix({xlUnsigned, 4, 0}, 10), ...
      |                        xfix({xlUnsigned, xl_nbits(linearAddr), 0}, 23))
      |     sm_TRIG_IN_CONF_1_en = true;
      | else
      |     sm_TRIG_IN_CONF_1_en = false;
      | end
      | 
      | 
      | % 'din' ports of 'To FIFO' blocks
      | 
      | 
      | % 'we' ports of 'To FIFO' blocks
      | 
      | 
      | % 'din' ports of 'To Register' blocks
      | sm_RSSI_PKT_DET_CONFIG_din = xl_force(xl_slice(wrDBus, 32 - 1, 0), ...
      |                                  xlUnsigned, ...
      |                                  0);
      | sm_TRIG_IN_CONF_6_din = xl_force(xl_slice(wrDBus, 32 - 1, 0), ...
      |                                  xlUnsigned, ...
      |                                  0);
      | sm_TRIG_IN_CONF_5_din = xl_force(xl_slice(wrDBus, 32 - 1, 0), ...
      |                                  xlUnsigned, ...
      |                                  0);
      | sm_TRIG_IN_CONF_4_din = xl_force(xl_slice(wrDBus, 32 - 1, 0), ...
      |                                  xlUnsigned, ...
      |                                  0);
      | sm_TRIG_IN_CONF_3_din = xl_force(xl_slice(wrDBus, 32 - 1, 0), ...
      |                                  xlUnsigned, ...
      |                                  0);
      | sm_TRIG_IN_CONF_2_din = xl_force(xl_slice(wrDBus, 32 - 1, 0), ...
      |                                  xlUnsigned, ...
      |                                  0);
      | sm_TRIG_IN_CONF_0_din = xl_force(xl_slice(wrDBus, 32 - 1, 0), ...
      |                                  xlUnsigned, ...
      |                                  0);
      | sm_TRIG_IN_CONF_8_din = xl_force(xl_slice(wrDBus, 32 - 1, 0), ...
      |                                  xlUnsigned, ...
      |                                  0);
      | sm_TRIG_IN_CONF_7_din = xl_force(xl_slice(wrDBus, 32 - 1, 0), ...
      |                                  xlUnsigned, ...
      |                                  0);
      | sm_TRIG_OUT_5_CONF_0_din = xl_force(xl_slice(wrDBus, 32 - 1, 0), ...
      |                                  xlUnsigned, ...
      |                                  0);
      | sm_TRIG_OUT_5_CONF_1_din = xl_force(xl_slice(wrDBus, 32 - 1, 0), ...
      |                                  xlUnsigned, ...
      |                                  0);
      | sm_TRIG_OUT_4_CONF_0_din = xl_force(xl_slice(wrDBus, 32 - 1, 0), ...
      |                                  xlUnsigned, ...
      |                                  0);
      | sm_TRIG_OUT_0_CONF_0_din = xl_force(xl_slice(wrDBus, 32 - 1, 0), ...
      |                                  xlUnsigned, ...
      |                                  0);
      | sm_TRIG_OUT_4_CONF_1_din = xl_force(xl_slice(wrDBus, 32 - 1, 0), ...
      |                                  xlUnsigned, ...
      |                                  0);
      | sm_TRIG_OUT_3_CONF_0_din = xl_force(xl_slice(wrDBus, 32 - 1, 0), ...
      |                                  xlUnsigned, ...
      |                                  0);
      | sm_TRIG_OUT_3_CONF_1_din = xl_force(xl_slice(wrDBus, 32 - 1, 0), ...
      |                                  xlUnsigned, ...
      |                                  0);
      | sm_TRIG_OUT_2_CONF_0_din = xl_force(xl_slice(wrDBus, 32 - 1, 0), ...
      |                                  xlUnsigned, ...
      |                                  0);
      | sm_TRIG_OUT_2_CONF_1_din = xl_force(xl_slice(wrDBus, 32 - 1, 0), ...
      |                                  xlUnsigned, ...
      |                                  0);
      | sm_TRIG_OUT_1_CONF_0_din = xl_force(xl_slice(wrDBus, 32 - 1, 0), ...
      |                                  xlUnsigned, ...
      |                                  0);
      | sm_TRIG_OUT_1_CONF_1_din = xl_force(xl_slice(wrDBus, 32 - 1, 0), ...
      |                                  xlUnsigned, ...
      |                                  0);
      | sm_TRIG_OUT_0_CONF_1_din = xl_force(xl_slice(wrDBus, 32 - 1, 0), ...
      |                                  xlUnsigned, ...
      |                                  0);
      | sm_RSSI_PKT_DET_DURATIONS_din = xl_force(xl_slice(wrDBus, 32 - 1, 0), ...
      |                                  xlUnsigned, ...
      |                                  0);
      | sm_RSSI_PKT_DET_THRESHOLDS_din = xl_force(xl_slice(wrDBus, 32 - 1, 0), ...
      |                                  xlUnsigned, ...
      |                                  0);
      | sm_TRIG_IN_CONF_1_din = xl_force(xl_slice(wrDBus, 32 - 1, 0), ...
      |                                  xlUnsigned, ...
      |                                  0);
      | 
      | 
      | persistent read_bank_out_reg; read_bank_out_reg = xl_state(0, {xlUnsigned, 32, 0});
      | read_bank_out = read_bank_out_reg;
      | 
      | persistent bankAddr_reg; bankAddr_reg = xl_state(0, bankAddr);
      | 
      | if bankAddr_reg == 0
      |     % Bank 0: Shared Memories
      |     read_bank_out_reg = 0;
      | elseif bankAddr_reg == 1
      |     % Bank 1: From/To FIFOs
      |     read_bank_out_reg =  0;
      | elseif bankAddr_reg == 2
      |     % Bank 2: From/To Registers
      |     read_bank_out_reg = reg_bank_out;
      | elseif bankAddr_reg == 3
      |     % Bank 3: Configuration Registers
      |     read_bank_out_reg = 0;
      | end
      | 
      | bankAddr_reg = bankAddr;
  sg_plb_addrpref : xbsIndex_r4/Gateway In  gui_display_data_type=Fixed-point  arith_type=Unsigned  n_bits=20  bin_pt=0  preci_type=Single  exp_width=8  frac_width=24  quantization="Round  (unbiased: +/- Inf)"  overflow=Saturate  period=xlGetNormalizedPeriod()  dbl_ovrd=off  timing_constraint=None  locs_specified=off  LOCs={}  UseAsADC=off  ADCChannel='1'  inherit_from_input=off  hdl_port=on  block_type=gatewayin
      settings: sginterface={'Xilinx'=>{'jtaghwcosim'=>{'non_memory_mapped_port'=>'sg_plb_addrpref'}},'iopad'=>{'constraint'=>'#'}}
  wires:
  plb_decode/2 -> plb_memmap/5, Sl_addrAck/1  "Sl_addrAck"
  plb_decode/4 -> Sl_wrDAck/1, Sl_wrComp/1  "Sl_wrDAck"
  plb_memmap/49 -> To Register23/2  "TRIG_IN_CONF_1_en"
  plb_memmap/48 -> To Register23/1  "TRIG_IN_CONF_1_din"
  plb_memmap/47 -> To Register22/2  "RSSI_PKT_DET_THRESHOLDS_en"
  plb_memmap/46 -> To Register22/1  "RSSI_PKT_DET_THRESHOLDS_din"
  plb_memmap/45 -> To Register21/2  "RSSI_PKT_DET_DURATIONS_en"
  plb_memmap/44 -> To Register21/1  "RSSI_PKT_DET_DURATIONS_din"
  plb_memmap/43 -> To Register20/2  "TRIG_OUT_0_CONF_1_en"
  plb_memmap/42 -> To Register20/1  "TRIG_OUT_0_CONF_1_din"
  plb_memmap/41 -> To Register19/2  "TRIG_OUT_1_CONF_1_en"
  plb_memmap/40 -> To Register19/1  "TRIG_OUT_1_CONF_1_din"
  plb_memmap/39 -> To Register18/2  "TRIG_OUT_1_CONF_0_en"
  plb_memmap/38 -> To Register18/1  "TRIG_OUT_1_CONF_0_din"
  plb_memmap/37 -> To Register17/2  "TRIG_OUT_2_CONF_1_en"
  plb_memmap/36 -> To Register17/1  "TRIG_OUT_2_CONF_1_din"
  plb_memmap/35 -> To Register16/2  "TRIG_OUT_2_CONF_0_en"
  plb_memmap/34 -> To Register16/1  "TRIG_OUT_2_CONF_0_din"
  plb_memmap/33 -> To Register15/2  "TRIG_OUT_3_CONF_1_en"
  plb_memmap/32 -> To Register15/1  "TRIG_OUT_3_CONF_1_din"
  plb_memmap/31 -> To Register14/2  "TRIG_OUT_3_CONF_0_en"
  plb_memmap/30 -> To Register14/1  "TRIG_OUT_3_CONF_0_din"
  plb_memmap/29 -> To Register13/2  "TRIG_OUT_4_CONF_1_en"
  plb_memmap/28 -> To Register13/1  "TRIG_OUT_4_CONF_1_din"
  plb_memmap/27 -> To Register12/2  "TRIG_OUT_0_CONF_0_en"
  plb_memmap/26 -> To Register12/1  "TRIG_OUT_0_CONF_0_din"
  plb_memmap/25 -> To Register11/2  "TRIG_OUT_4_CONF_0_en"
  plb_memmap/24 -> To Register11/1  "TRIG_OUT_4_CONF_0_din"
  plb_memmap/23 -> To Register10/2  "TRIG_OUT_5_CONF_1_en"
  plb_memmap/22 -> To Register10/1  "TRIG_OUT_5_CONF_1_din"
  plb_memmap/21 -> To Register9/2  "TRIG_OUT_5_CONF_0_en"
  plb_memmap/20 -> To Register9/1  "TRIG_OUT_5_CONF_0_din"
  plb_memmap/19 -> To Register8/2  "TRIG_IN_CONF_7_en"
  plb_memmap/18 -> To Register8/1  "TRIG_IN_CONF_7_din"
  plb_memmap/17 -> To Register7/2  "TRIG_IN_CONF_8_en"
  plb_memmap/16 -> To Register7/1  "TRIG_IN_CONF_8_din"
  plb_memmap/15 -> To Register6/2  "TRIG_IN_CONF_0_en"
  plb_memmap/14 -> To Register6/1  "TRIG_IN_CONF_0_din"
  plb_memmap/13 -> To Register5/2  "TRIG_IN_CONF_2_en"
  plb_memmap/12 -> To Register5/1  "TRIG_IN_CONF_2_din"
  plb_memmap/11 -> To Register4/2  "TRIG_IN_CONF_3_en"
  plb_memmap/10 -> To Register4/1  "TRIG_IN_CONF_3_din"
  plb_memmap/9 -> To Register3/2  "TRIG_IN_CONF_4_en"
  plb_memmap/8 -> To Register3/1  "TRIG_IN_CONF_4_din"
  plb_memmap/7 -> To Register2/2  "TRIG_IN_CONF_5_en"
  plb_memmap/6 -> To Register2/1  "TRIG_IN_CONF_5_din"
  plb_memmap/5 -> To Register1/2  "TRIG_IN_CONF_6_en"
  plb_memmap/4 -> To Register1/1  "TRIG_IN_CONF_6_din"
  plb_memmap/3 -> To Register/2  "RSSI_PKT_DET_CONFIG_en"
  plb_memmap/2 -> To Register/1  "RSSI_PKT_DET_CONFIG_din"
  plb_memmap/1 -> plb_decode/6  "rdData"
  To Register23/1 -> plb_memmap/31  "TRIG_IN_CONF_1_dout"
  To Register22/1 -> plb_memmap/30  "RSSI_PKT_DET_THRESHOLDS_dout"
  To Register21/1 -> plb_memmap/29  "RSSI_PKT_DET_DURATIONS_dout"
  To Register20/1 -> plb_memmap/28  "TRIG_OUT_0_CONF_1_dout"
  To Register19/1 -> plb_memmap/27  "TRIG_OUT_1_CONF_1_dout"
  To Register18/1 -> plb_memmap/26  "TRIG_OUT_1_CONF_0_dout"
  To Register17/1 -> plb_memmap/25  "TRIG_OUT_2_CONF_1_dout"
  To Register16/1 -> plb_memmap/24  "TRIG_OUT_2_CONF_0_dout"
  To Register15/1 -> plb_memmap/23  "TRIG_OUT_3_CONF_1_dout"
  To Register14/1 -> plb_memmap/22  "TRIG_OUT_3_CONF_0_dout"
  To Register13/1 -> plb_memmap/21  "TRIG_OUT_4_CONF_1_dout"
  To Register12/1 -> plb_memmap/20  "TRIG_OUT_0_CONF_0_dout"
  To Register11/1 -> plb_memmap/19  "TRIG_OUT_4_CONF_0_dout"
  To Register10/1 -> plb_memmap/18  "TRIG_OUT_5_CONF_1_dout"
  To Register9/1 -> plb_memmap/17  "TRIG_OUT_5_CONF_0_dout"
  To Register8/1 -> plb_memmap/16  "TRIG_IN_CONF_7_dout"
  To Register7/1 -> plb_memmap/15  "TRIG_IN_CONF_8_dout"
  To Register6/1 -> plb_memmap/14  "TRIG_IN_CONF_0_dout"
  To Register5/1 -> plb_memmap/13  "TRIG_IN_CONF_2_dout"
  To Register4/1 -> plb_memmap/12  "TRIG_IN_CONF_3_dout"
  To Register3/1 -> plb_memmap/11  "TRIG_IN_CONF_4_dout"
  To Register2/1 -> plb_memmap/10  "TRIG_IN_CONF_5_dout"
  To Register1/1 -> plb_memmap/9  "TRIG_IN_CONF_6_dout"
  To Register/1 -> plb_memmap/8  "RSSI_PKT_DET_CONFIG_dout"
  From Register1/1 -> plb_memmap/7  "TRIG_OUT_dout"
  From Register/1 -> plb_memmap/6  "CORE_INFO_dout"
  plb_decode/6 -> plb_memmap/4  "RNWReg"
  plb_decode/9 -> plb_memmap/3  "linearAddr"
  plb_decode/5 -> plb_memmap/2  "bankAddr"
  plb_decode/1 -> plb_memmap/1  "wrDBusReg"
  plb_decode/8 -> Sl_rdDBus/1  "Sl_rdDBus"
  plb_decode/7 -> Sl_rdDAck/1  "Sl_rdDAck"
  plb_decode/3 -> Sl_rdComp/1  "Sl_rdComp"
  sg_plb_addrpref/1 -> plb_decode/7  "addrPref"
  PLB_wrDBus/1 -> plb_decode/5  "PLB_wrDBus"
  PLB_RNW/1 -> plb_decode/4  "PLB_RNW"
  PLB_PAValid/1 -> plb_decode/3  "PLB_PAValid"
  PLB_ABus/1 -> plb_decode/2  "PLB_ABus"
  SPLB_Rst/1 -> plb_decode/1  "SPLB_Rst"
  Constant6/1 -> sg_plb_addrpref/1
  Constant5/1 -> Sl_wait/1  "Sl_wait"
  Constant4/1 -> PLB_wrDBus/1
  Constant3/1 -> PLB_RNW/1
  Constant2/1 -> PLB_PAValid/1
  Constant1/1 -> PLB_ABus/1
  Constant/1 -> SPLB_Rst/1
  Sl_wrComp/1 -> Terminator6/1
  Sl_wrDAck/1 -> Terminator5/1
  Sl_wait/1 -> Terminator4/1
  Sl_rdDBus/1 -> Terminator3/1
  Sl_rdDAck/1 -> Terminator2/1
  Sl_rdComp/1 -> Terminator1/1
  Sl_addrAck/1 -> Terminator/1

== system w2_warplab_trigger_proc/Posedge ==
  note: Rising Edge Detection
  D : Inport
  Delay : xbsIndex_r4/Delay  rst=off  infoeditControl=Selection of Reset will increase slice count due to use of real FFs and instead of SRLs  en=off  latency=1  dbl_ovrd=off  reg_retiming=off  block_type=delay
      settings: infoedit=Hardware notes: A delay line is a chain, each link of which is an SRL16 followed by a flip-flop. If register retiming is enabled, the delay line is a chain of flip-flops.  xl_area=[1 1 0 0 0 0 0]  block_version=VER_STRING_GOES_HERE
  Inverter : xbsIndex_r4/Inverter  en=off  latency=0  dbl_ovrd=off  block_type=inv
      settings: xl_area=[0 0 0 0 0 0 0]  block_version=VER_STRING_GOES_HERE
  Logical1 : xbsIndex_r4/Logical  logical_function=AND  inputs=2  en=off  latency=0  precision=Full  arith_type=Unsigned  n_bits=8  bin_pt=2  align_bp=on  dbl_ovrd=off  block_type=logical
      settings: xl_area=[1 0 0 1 0 0 0]  block_version=VER_STRING_GOES_HERE
  Q : Outport
  wires:
  D/1 -> Logical1/2, Delay/1
  Logical1/1 -> Q/1
  Inverter/1 -> Logical1/1
  Delay/1 -> Inverter/1
